simulink model "model"  (Simulink 7.5)
settings: Solver=ode45  StartTime=0.0  StopTime=100  RelTol=1e-3
values from neighbouring files (symbols this model uses):
  G = 33    [model_sim.m]
settings Model: Creator=303-t  LastModifiedBy=Michael
settings DataIOCC: OutputSaveName=xout

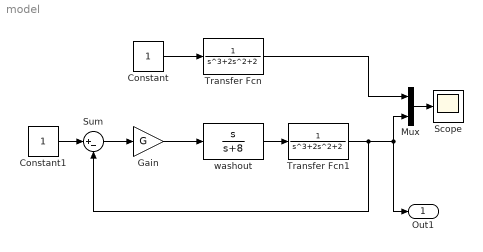
== system model ==
  Constant : Constant
  Constant1 : Constant
  Gain : Gain  Gain=G
  Mux : Mux  Inputs=2
  Scope : Scope
  Sum : Sum  Inputs=|+-
  Transfer Fcn : TransferFcn  Denominator=[1 2 0 2]
  Transfer Fcn1 : TransferFcn  Denominator=[1 2 0 2]
  washout : TransferFcn  Numerator=[1 0]  Denominator=[1 8]
  Out1 : Outport
  wires:
  Constant/1 -> Transfer Fcn/1
  Constant1/1 -> Sum/1
  Sum/1 -> Gain/1
  Gain/1 -> washout/1
  washout/1 -> Transfer Fcn1/1
  Transfer Fcn1/1 -> Sum/2, Mux/2, Out1/1
  Mux/1 -> Scope/1
  Transfer Fcn/1 -> Mux/1
